simulink library "BEML_EMU_DoorsInput_Lib"  (R2019b)
settings: Solver=VariableStepAuto  StartTime=0.0  StopTime=10.0  RelTol=1e-3
undefined symbols (not defined in the file): DoorsSampleTime, DoorWinder, ElectricalSignals, EmerDoorLatched, EmerDoorOpenFault, EmergencyDoorGasSpring, EmergencyDoorHandle, EmergencyDoorMechanicalUnlocked, HasCab, InputControlStates, RampCoverLockingLever, RampHandle, RampMiddleSupport, RampWinder
libraries: simulink x128, $bdroot x8, VectorOperationsLib x1
(part 1 of 2)
settings Model: Creator=rleighton  LastModifiedBy=bnadpurohit
settings DataIOCC: ReturnWorkspaceOutputs=off
settings DebuggingCC: ArithmeticOperatorsInVariantConditions=warning
settings SFSimCC: SimUseLocalCustomCode=off  CustomCodeUndefinedFunction=UseInterfaceOnly
settings RTWCC: RTWUseLocalCustomCode=off

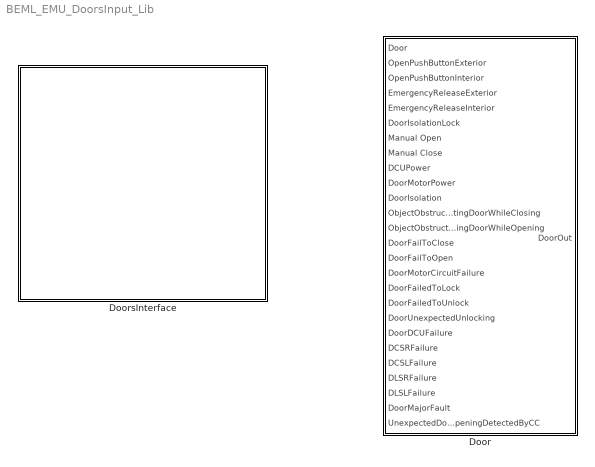
== system BEML_EMU_DoorsInput_Lib ==
  Door : Subsystem  mask{isLeft=on}
  DoorsInterface : Subsystem  SystemSampleTime=0.001

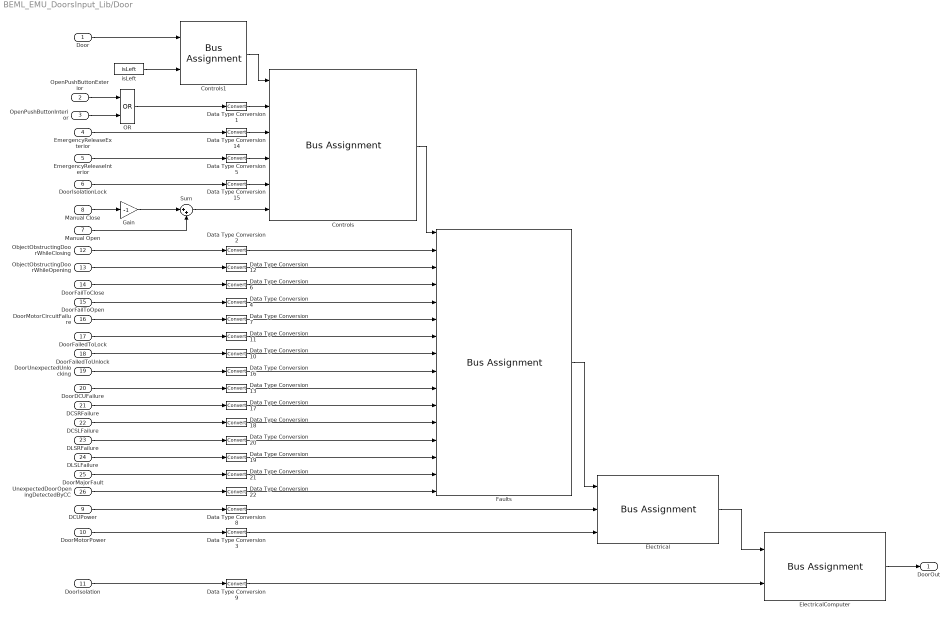
== system BEML_EMU_DoorsInput_Lib/Door ==
  Door : Inport
  OpenPushButtonExterior : Inport  Port=2
  OpenPushButtonInterior : Inport  Port=3
  EmergencyReleaseExterior : Inport  Port=4
  EmergencyReleaseInterior : Inport  Port=5
  DoorIsolationLock : Inport  Port=6
  Manual Open : Inport  Port=7
  Manual Close : Inport  Port=8
  DCUPower : Inport  Port=9
  DoorMotorPower : Inport  Port=10
  DoorIsolation : Inport  Port=11
  ObjectObstructingDoorWhileClosing : Inport  Port=12
  ObjectObstructingDoorWhileOpening : Inport  Port=13
  DoorFailToClose : Inport  Port=14
  DoorFailToOpen : Inport  Port=15
  DoorMotorCircuitFailure : Inport  Port=16
  DoorFailedToLock : Inport  Port=17
  DoorFailedToUnlock : Inport  Port=18
  DoorUnexpectedUnlocking : Inport  Port=19
  DoorDCUFailure : Inport  Port=20
  DCSRFailure : Inport  Port=21
  DCSLFailure : Inport  Port=22
  DLSRFailure : Inport  Port=23
  DLSLFailure : Inport  Port=24
  DoorMajorFault : Inport  Port=25
  UnexpectedDoorOpeningDetectedByCC : Inport  Port=26
  Controls : BusAssignment  AssignedSignals=InputControlStates.LocalDoorOpenPB,InputControlStates.EmergencyAccessDevice,InputControlStates.EmergencyEgressDevice,InputControlStates.LocalDoorIsolationLock,InputControlStates.OpenCloseWidget
  Controls1 : BusAssignment  AssignedSignals=Config.isLeft
  Data Type Conversion{1..22} (22 alike) : DataTypeConversion
  Electrical : BusAssignment  AssignedSignals=ElectricalSignals.DoorControlPower,ElectricalSignals.DoorMotorPower
  ElectricalComputer : BusAssignment  AssignedSignals=ElectricalSignals.DoorIsolation
  Faults : BusAssignment  AssignedSignals=Faults.ObjectObstructingDoorWhileClosing,Faults.ObjectObstructingDoorWhileOpening,Faults.DoorFailToClose,Faults.DoorFailToOpen,Faults.DoorMotorCircuitFailure,Faults.DoorFailedToLock,Faults.DoorFailedToUnlock,Faults.DoorUnexpectedUnlocking,Faults.DoorDCUFailure,Faults.DCSRFailure,Faults.DCSLFailure,Faults.DLSRFailure,Faults.DLSLFailure,Faults.DoorMajorFault,Faults.UnexpectedDoorOpeningDetectedByCC
  Gain : Gain  Gain=-1
  OR : Logic  Operator=OR  AllPortsSameDT=off  OutDataTypeStr=boolean
  Sum : Sum  Inputs=|++
  isLeft : Constant  Value=isLeft
  "DoorOut " : Outport  VectorParamsAs1DForOutWhenUnconnected=off
  wires:
  Data Type Conversion22/1 -> Faults/16
  UnexpectedDoorOpeningDetectedByCC/1 -> Data Type Conversion22/1
  OR/1 -> Data Type Conversion1/1
  OpenPushButtonInterior/1 -> OR/2
  DoorIsolationLock/1 -> Data Type Conversion15/1
  EmergencyReleaseExterior/1 -> Data Type Conversion14/1
  ObjectObstructingDoorWhileOpening/1 -> Data Type Conversion12/1
  Data Type Conversion12/1 -> Faults/3
  Data Type Conversion8/1 -> Electrical/2
  Data Type Conversion1/1 -> Controls/2
  OpenPushButtonExterior/1 -> OR/1
  Electrical/1 -> ElectricalComputer/1
  Sum/1 -> Controls/6
  ObjectObstructingDoorWhileClosing/1 -> Data Type Conversion2/1
  Data Type Conversion2/1 -> Faults/2
  Faults/1 -> Electrical/1
  Controls/1 -> Faults/1
  Door/1 -> Controls1/1
  Controls1/1 -> Controls/1
  isLeft/1 -> Controls1/2
  Manual Close/1 -> Gain/1
  Gain/1 -> Sum/1
  Manual Open/1 -> Sum/2
  DCUPower/1 -> Data Type Conversion8/1
  Data Type Conversion5/1 -> Controls/4
  Data Type Conversion15/1 -> Controls/5
  Data Type Conversion14/1 -> Controls/3
  DoorMotorPower/1 -> Data Type Conversion3/1
  Data Type Conversion3/1 -> Electrical/3
  Data Type Conversion6/1 -> Faults/4
  DoorFailToClose/1 -> Data Type Conversion6/1
  Data Type Conversion4/1 -> Faults/5
  DoorFailToOpen/1 -> Data Type Conversion4/1
  DoorMotorCircuitFailure/1 -> Data Type Conversion7/1
  Data Type Conversion7/1 -> Faults/6
  ElectricalComputer/1 -> "DoorOut "/1
  Data Type Conversion9/1 -> ElectricalComputer/2
  DoorIsolation/1 -> Data Type Conversion9/1
  Data Type Conversion17/1 -> Faults/11
  DCSRFailure/1 -> Data Type Conversion17/1
  DoorDCUFailure/1 -> Data Type Conversion13/1
  Data Type Conversion13/1 -> Faults/10
  DoorUnexpectedUnlocking/1 -> Data Type Conversion16/1
  Data Type Conversion16/1 -> Faults/9
  Data Type Conversion11/1 -> Faults/7
  DoorFailedToLock/1 -> Data Type Conversion11/1
  Data Type Conversion10/1 -> Faults/8
  DoorFailedToUnlock/1 -> Data Type Conversion10/1
  DCSLFailure/1 -> Data Type Conversion18/1
  Data Type Conversion18/1 -> Faults/12
  Data Type Conversion20/1 -> Faults/13
  DLSRFailure/1 -> Data Type Conversion20/1
  Data Type Conversion19/1 -> Faults/14
  DLSLFailure/1 -> Data Type Conversion19/1
  DoorMajorFault/1 -> Data Type Conversion21/1
  Data Type Conversion21/1 -> Faults/15
  EmergencyReleaseInterior/1 -> Data Type Conversion5/1

== system BEML_EMU_DoorsInput_Lib/DoorsInterface ==
  DoorsInputAdapter : Subsystem  TreatAsAtomicUnit=on  SystemSampleTime=DoorsSampleTime

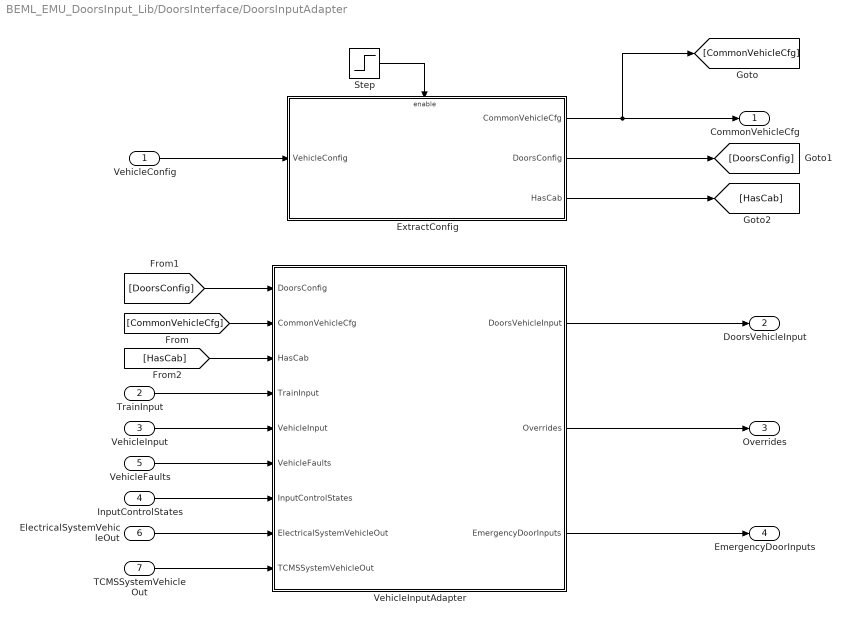
== system BEML_EMU_DoorsInput_Lib/DoorsInterface/DoorsInputAdapter ==
  VehicleConfig : Inport  SampleTime=0.05
  TrainInput : Inport  Port=2  SampleTime=0.05
  VehicleInput : Inport  Port=3  SampleTime=0.05
  InputControlStates : Inport  Port=4  SampleTime=0.05
  VehicleFaults : Inport  Port=5  SampleTime=0.05
  ElectricalSystemVehicleOut : Inport  Port=6  SampleTime=0.05
  TCMSSystemVehicleOut : Inport  Port=7  SampleTime=0.05
  ExtractConfig : Subsystem
  Step : Step  Before=1  After=0
  VehicleInputAdapter : Subsystem
  CommonVehicleCfg : Outport  VectorParamsAs1DForOutWhenUnconnected=off
  DoorsVehicleInput : Outport  Port=2  VectorParamsAs1DForOutWhenUnconnected=off
  Overrides : Outport  Port=3  VectorParamsAs1DForOutWhenUnconnected=off
  EmergencyDoorInputs : Outport  Port=4  VectorParamsAs1DForOutWhenUnconnected=off
  wires:
  [HasCab] -> VehicleInputAdapter/3(HasCab)
  ExtractConfig/3(HasCab) -> [HasCab]
  [CommonVehicleCfg] -> VehicleInputAdapter/2(CommonVehicleCfg)
  VehicleInputAdapter/3(EmergencyDoorInputs) -> EmergencyDoorInputs/1
  [DoorsConfig] -> VehicleInputAdapter/1(DoorsConfig)
  ExtractConfig/2(DoorsConfig) -> [DoorsConfig]
  InputControlStates/1 -> VehicleInputAdapter/7(InputControlStates)
  VehicleConfig/1 -> ExtractConfig/1(VehicleConfig)
  VehicleFaults/1 -> VehicleInputAdapter/6(VehicleFaults)
  TrainInput/1 -> VehicleInputAdapter/4(TrainInput)
  VehicleInput/1 -> VehicleInputAdapter/5(VehicleInput)
  ElectricalSystemVehicleOut/1 -> VehicleInputAdapter/8(ElectricalSystemVehicleOut)
  TCMSSystemVehicleOut/1 -> VehicleInputAdapter/9(TCMSSystemVehicleOut)
  ExtractConfig/1(CommonVehicleCfg) -> [CommonVehicleCfg], CommonVehicleCfg/1
  Step/1 -> ExtractConfig/Enable
  VehicleInputAdapter/1(DoorsVehicleInput) -> DoorsVehicleInput/1
  VehicleInputAdapter/2(Overrides) -> Overrides/1

== system BEML_EMU_DoorsInput_Lib/DoorsInterface/DoorsInputAdapter/ExtractConfig ==
  VehicleConfig : Inport
  Enable : EnablePort
  ExtractConfig : Subsystem
  CommonVehicleCfg : Outport  VectorParamsAs1DForOutWhenUnconnected=off
  DoorsConfig : Outport  Port=2  VectorParamsAs1DForOutWhenUnconnected=off
  HasCab : Outport  Port=3  VectorParamsAs1DForOutWhenUnconnected=off
  wires:
  ExtractConfig/3(HasCab) -> HasCab/1
  ExtractConfig/2(DoorsConfig) -> DoorsConfig/1
  ExtractConfig/1(CommonVehicleConfig) -> CommonVehicleCfg/1
  VehicleConfig/1 -> ExtractConfig/1(VehicleConfig)

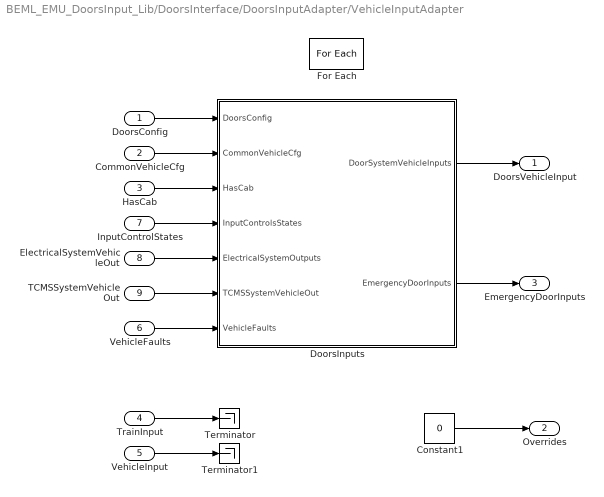
== system BEML_EMU_DoorsInput_Lib/DoorsInterface/DoorsInputAdapter/VehicleInputAdapter ==
  DoorsConfig : Inport  Partition=on  PartitionDimension=1  PartitionWidth=1  PartitionOffset=0
  CommonVehicleCfg : Inport  Port=2  Partition=on  PartitionDimension=1  PartitionWidth=1  PartitionOffset=0
  HasCab : Inport  Port=3  Partition=on  PartitionDimension=1  PartitionWidth=1  PartitionOffset=0
  TrainInput : Inport  Port=4
  VehicleInput : Inport  Port=5  Partition=on  PartitionDimension=1  PartitionWidth=1  PartitionOffset=0
  VehicleFaults : Inport  Port=6  Partition=on  PartitionDimension=1  PartitionWidth=1  PartitionOffset=0
  InputControlStates : Inport  Port=7  Partition=on  PartitionDimension=1  PartitionWidth=1  PartitionOffset=0
  ElectricalSystemVehicleOut : Inport  Port=8  Partition=on  PartitionDimension=1  PartitionWidth=1  PartitionOffset=0
  TCMSSystemVehicleOut : Inport  Port=9  Partition=on  PartitionDimension=1  PartitionWidth=1  PartitionOffset=0
  Constant1 : Constant  Value=0  OutDataTypeStr=Bus: BD_DoorSystem_In_Overrides
  DoorsInputs : Subsystem
  For Each : ForEach  DisableCoverage=on
  Terminator : Terminator
  Terminator1 : Terminator
  DoorsVehicleInput : Outport  ConcatenationDimension=1  VectorParamsAs1DForOutWhenUnconnected=off
  Overrides : Outport  Port=2  ConcatenationDimension=1  VectorParamsAs1DForOutWhenUnconnected=off
  EmergencyDoorInputs : Outport  Port=3  ConcatenationDimension=1  VectorParamsAs1DForOutWhenUnconnected=off
  wires:
  HasCab/1 -> DoorsInputs/3(HasCab)
  CommonVehicleCfg/1 -> DoorsInputs/2(CommonVehicleCfg)
  DoorsInputs/2(EmergencyDoorInputs) -> EmergencyDoorInputs/1
  DoorsConfig/1 -> DoorsInputs/1(DoorsConfig)
  InputControlStates/1 -> DoorsInputs/4(InputControlsStates)
  Constant1/1 -> Overrides/1
  DoorsInputs/1(DoorSystemVehicleInputs) -> DoorsVehicleInput/1
  TCMSSystemVehicleOut/1 -> DoorsInputs/6(TCMSSystemVehicleOut)
  ElectricalSystemVehicleOut/1 -> DoorsInputs/5(ElectricalSystemOutputs)
  VehicleFaults/1 -> DoorsInputs/7(VehicleFaults)
  VehicleInput/1 -> Terminator1/1
  TrainInput/1 -> Terminator/1

== system BEML_EMU_DoorsInput_Lib/DoorsInterface/DoorsInputAdapter/ExtractConfig/ExtractConfig ==
  VehicleConfig : Inport  Partition=on  PartitionDimension=1  PartitionWidth=1  PartitionOffset=0  BusOutputAsStruct=on
  Bus Selector : BusSelector  OutputSignals=Common,Doors,Equipment.HasCab
  For Each : ForEach  DisableCoverage=on
  CommonVehicleConfig : Outport  ConcatenationDimension=1  VectorParamsAs1DForOutWhenUnconnected=off
  DoorsConfig : Outport  Port=2  ConcatenationDimension=1  VectorParamsAs1DForOutWhenUnconnected=off
  HasCab : Outport  Port=3  ConcatenationDimension=1  VectorParamsAs1DForOutWhenUnconnected=off
  wires:
  Bus Selector/3 -> HasCab/1  "<HasCab>"
  Bus Selector/2 -> DoorsConfig/1  "<Doors>"
  VehicleConfig/1 -> Bus Selector/1
  Bus Selector/1 -> CommonVehicleConfig/1  "<Common>"

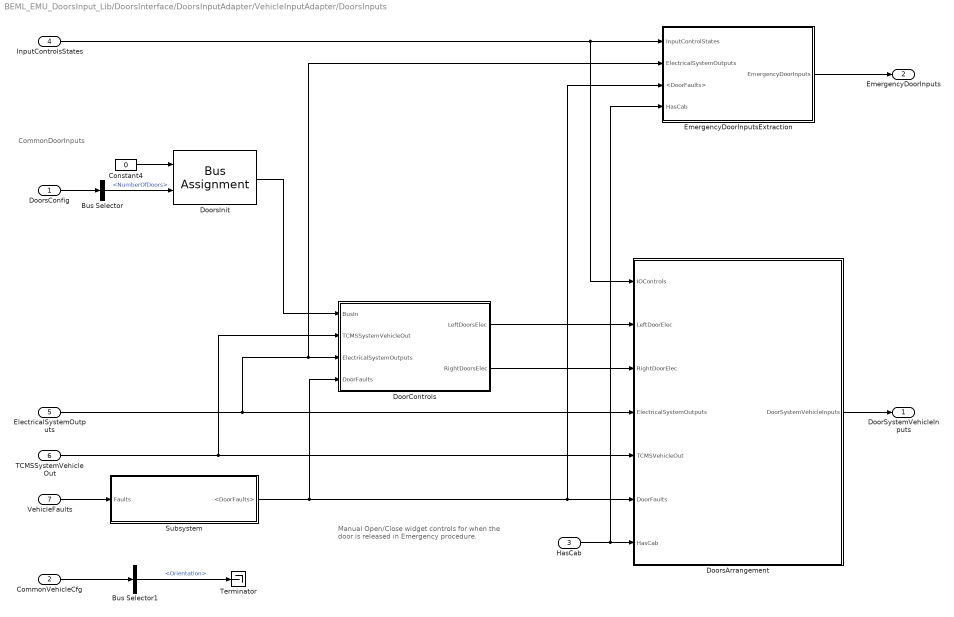
== system BEML_EMU_DoorsInput_Lib/DoorsInterface/DoorsInputAdapter/VehicleInputAdapter/DoorsInputs ==
  note: CommonDoorInputs
  note: Manual Open/Close widget controls for when the door is released in Emergency procedure.
  DoorsConfig : Inport
  CommonVehicleCfg : Inport  Port=2
  HasCab : Inport  Port=3
  InputControlsStates : Inport  Port=4
  ElectricalSystemOutputs : Inport  Port=5
  TCMSSystemVehicleOut : Inport  Port=6
  VehicleFaults : Inport  Port=7
  Bus Selector : BusSelector  OutputSignals=NumberOfDoors
  Bus Selector1 : BusSelector  OutputSignals=Orientation
  Constant4 : Constant  Value=0  OutDataTypeStr=Bus: BD_DoorSystem_In_Door  SampleTime=-1
  DoorControls : Subsystem
  DoorsArrangement : Subsystem
  DoorsInit : BusAssignment  AssignedSignals=Config.NumberOfDoors
  EmergencyDoorInputsExtraction : Subsystem
  Subsystem : Subsystem
  Terminator : Terminator
  DoorSystemVehicleInputs : Outport  VectorParamsAs1DForOutWhenUnconnected=off
  EmergencyDoorInputs : Outport  Port=2  VectorParamsAs1DForOutWhenUnconnected=off
  wires:
  HasCab/1 -> DoorsArrangement/7(HasCab), EmergencyDoorInputsExtraction/4(HasCab)
  DoorControls/2(RightDoorsElec) -> DoorsArrangement/3(RightDoorElec)
  Bus Selector1/1 -> Terminator/1  "<Orientation>"
  Subsystem/1(<DoorFaults>) -> DoorsArrangement/6(DoorFaults), EmergencyDoorInputsExtraction/3(<DoorFaults>), DoorControls/4(DoorFaults)
  VehicleFaults/1 -> Subsystem/1(Faults)
  CommonVehicleCfg/1 -> Bus Selector1/1
  EmergencyDoorInputsExtraction/1(EmergencyDoorInputs) -> EmergencyDoorInputs/1
  InputControlsStates/1 -> DoorsArrangement/1(IOControls), EmergencyDoorInputsExtraction/1(InputControlStates)
  ElectricalSystemOutputs/1 -> DoorsArrangement/4(ElectricalSystemOutputs), DoorControls/3(ElectricalSystemOutputs), EmergencyDoorInputsExtraction/2(ElectricalSystemOutputs)
  DoorsConfig/1 -> Bus Selector/1
  DoorControls/1(LeftDoorsElec) -> DoorsArrangement/2(LeftDoorElec)
  TCMSSystemVehicleOut/1 -> DoorsArrangement/5(TCMSVehicleOut), DoorControls/2(TCMSSystemVehicleOut)
  Bus Selector/1 -> DoorsInit/2  "<NumberOfDoors>"
  DoorsInit/1 -> DoorControls/1(BusIn)
  DoorsArrangement/1(DoorSystemVehicleInputs) -> DoorSystemVehicleInputs/1
  Constant4/1 -> DoorsInit/1

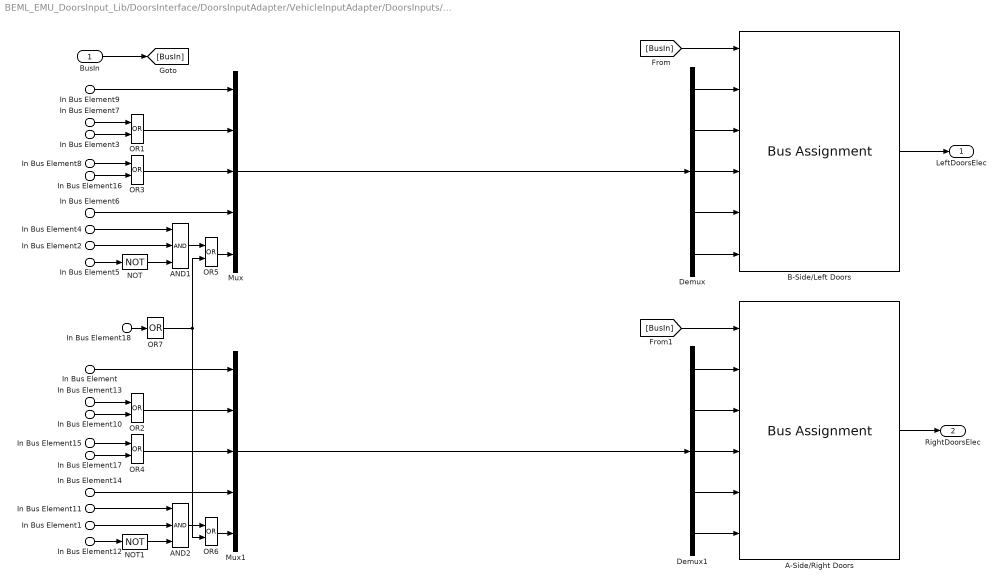
== system BEML_EMU_DoorsInput_Lib/DoorsInterface/DoorsInputAdapter/VehicleInputAdapter/DoorsInputs/DoorControls ==
  BusIn : Inport
  In Bus Element6 : Inport  Port=2  PortName=TCMSSystemVehicleOut  Element=Control.DoorSystem.LeftDoorEmergencyRelease
  In Bus Element7 : Inport  Port=2  PortName=TCMSSystemVehicleOut  Element=Control.DoorSystem.LeftSideDoorOpenRequest
  In Bus Element8 : Inport  Port=2  PortName=TCMSSystemVehicleOut  Element=Control.DoorSystem.LeftSideDoorCloseRequest
  In Bus Element9 : Inport  Port=2  PortName=TCMSSystemVehicleOut  Element=Control.DoorSystem.LeftSideDoorRelease
  In Bus Element : Inport  Port=2  PortName=TCMSSystemVehicleOut  Element=Control.DoorSystem.RightSideDoorRelease
  In Bus Element13 : Inport  Port=2  PortName=TCMSSystemVehicleOut  Element=Control.DoorSystem.RightSideDoorOpenRequest
  In Bus Element14 : Inport  Port=2  PortName=TCMSSystemVehicleOut  Element=Control.DoorSystem.RightDoorEmergencyRelease
  In Bus Element15 : Inport  Port=2  PortName=TCMSSystemVehicleOut  Element=Control.DoorSystem.RightSideDoorCloseRequest
  In Bus Element2 : Inport  Port=3  PortName=ElectricalSystemOutputs  Element=Doors.ZeroSpeed
  In Bus Element1 : Inport  Port=3  PortName=ElectricalSystemOutputs  Element=Doors.ZeroSpeed
  In Bus Element3 : Inport  Port=3  PortName=ElectricalSystemOutputs  Element=Doors.LeftDoorOpenCmdInLimpHome
  In Bus Element4 : Inport  Port=3  PortName=ElectricalSystemOutputs  Element=Doors.LeftDoorEnable
  In Bus Element5 : Inport  Port=3  PortName=ElectricalSystemOutputs  Element=Doors.LeftHoldDoorClose
  In Bus Element10 : Inport  Port=3  PortName=ElectricalSystemOutputs  Element=Doors.RightDoorOpenCmdInLimpHome
  In Bus Element11 : Inport  Port=3  PortName=ElectricalSystemOutputs  Element=Doors.RightDoorEnable
  In Bus Element12 : Inport  Port=3  PortName=ElectricalSystemOutputs  Element=Doors.RightHoldDoorClose
  In Bus Element16 : Inport  Port=3  PortName=ElectricalSystemOutputs  Element=Doors.LeftDoorClose
  In Bus Element17 : Inport  Port=3  PortName=ElectricalSystemOutputs  Element=Doors.RightDoorClose
  In Bus Element18 : Inport  Port=4  PortName=DoorFaults  Element=UnexpectedDoorOpeningDetectedByCC
  A-Side/Right Doors : BusAssignment  AssignedSignals=ElectricalSignals.DoorRelease,ElectricalSignals.DoorOpen,ElectricalSignals.DoorClose,ElectricalSignals.DoorEmergencyRelease,ElectricalSignals.DoorEnable
  AND1 : Logic  Inputs=3  AllPortsSameDT=off  OutDataTypeStr=boolean
  AND2 : Logic  Inputs=3  AllPortsSameDT=off  OutDataTypeStr=boolean
  B-Side/Left Doors : BusAssignment  AssignedSignals=ElectricalSignals.DoorRelease,ElectricalSignals.DoorOpen,ElectricalSignals.DoorClose,ElectricalSignals.DoorEmergencyRelease,ElectricalSignals.DoorEnable
  Demux : Demux  Outputs=5
  Demux1 : Demux  Outputs=5
  Mux : Mux  Inputs=5
  Mux1 : Mux  Inputs=5
  NOT : Logic  Operator=NOT  AllPortsSameDT=off  OutDataTypeStr=boolean
  NOT1 : Logic  Operator=NOT  AllPortsSameDT=off  OutDataTypeStr=boolean
  OR{1..6} (6 alike) : Logic  Operator=OR  AllPortsSameDT=off  OutDataTypeStr=boolean
  OR7 : Logic  Operator=OR  Inputs=1  AllPortsSameDT=off  OutDataTypeStr=boolean
  LeftDoorsElec : Outport
  RightDoorsElec : Outport  Port=2
  wires:
  OR7/1 -> OR5/2, OR6/2
  In Bus Element18/1 -> OR7/1
  OR5/1 -> Mux/5
  OR6/1 -> Mux1/5
  NOT1/1 -> AND2/3
  NOT/1 -> AND1/3
  In Bus Element5/1 -> NOT/1
  In Bus Element12/1 -> NOT1/1
  In Bus Element17/1 -> OR4/2
  In Bus Element15/1 -> OR4/1
  In Bus Element16/1 -> OR3/2
  In Bus Element8/1 -> OR3/1
  Demux1/5 -> A-Side/Right Doors/6
  Demux1/4 -> A-Side/Right Doors/5
  Demux1/3 -> A-Side/Right Doors/4
  Demux1/2 -> A-Side/Right Doors/3
  Demux1/1 -> A-Side/Right Doors/2
  Demux/5 -> B-Side/Left Doors/6
  Demux/4 -> B-Side/Left Doors/5
  Demux/3 -> B-Side/Left Doors/4
  Demux/2 -> B-Side/Left Doors/3
  Demux/1 -> B-Side/Left Doors/2
  Mux1/1 -> Demux1/1
  Mux/1 -> Demux/1
  [BusIn] -> B-Side/Left Doors/1
  BusIn/1 -> [BusIn]
  In Bus Element/1 -> Mux1/1
  In Bus Element11/1 -> AND2/1
  In Bus Element13/1 -> OR2/1
  In Bus Element10/1 -> OR2/2
  A-Side/Right Doors/1 -> RightDoorsElec/1
  OR4/1 -> Mux1/3
  [BusIn] -> A-Side/Right Doors/1
  In Bus Element1/1 -> AND2/2
  AND2/1 -> OR6/1
  OR2/1 -> Mux1/2
  In Bus Element14/1 -> Mux1/4
  In Bus Element2/1 -> AND1/2
  In Bus Element4/1 -> AND1/1
  AND1/1 -> OR5/1
  In Bus Element3/1 -> OR1/2
  In Bus Element7/1 -> OR1/1
  OR1/1 -> Mux/2
  OR3/1 -> Mux/3
  In Bus Element9/1 -> Mux/1
  In Bus Element6/1 -> Mux/4
  B-Side/Left Doors/1 -> LeftDoorsElec/1

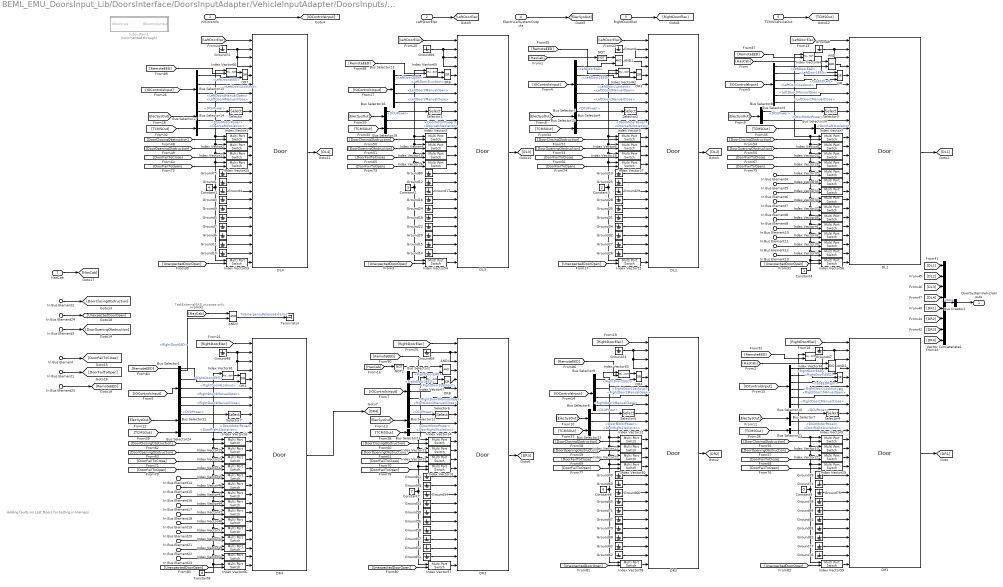
== system BEML_EMU_DoorsInput_Lib/DoorsInterface/DoorsInputAdapter/VehicleInputAdapter/DoorsInputs/DoorsArrangement ==
  note: Adding faults on Last Doors for testing in Harness
  note: TestExternalEAD purpose only
  IOControls : Inport
  LeftDoorElec : Inport  Port=2
  RightDoorElec : Inport  Port=3
  ElectricalSystemOutputs : Inport  Port=4
  TCMSVehicleOut : Inport  Port=5
  In Bus Element2 : Inport  Port=6  PortName=DoorFaults  Element=ObjectObstructingDoorWhileClosing
  In Bus Element3 : Inport  Port=6  PortName=DoorFaults  Element=ObjectObstructingDoorWhileOpening
  In Bus Element : Inport  Port=6  PortName=DoorFaults  Element=DoorFailToClose
  In Bus Element1 : Inport  Port=6  PortName=DoorFaults  Element=DoorFailToOpen
  In Bus Element4 : Inport  Port=6  PortName=DoorFaults  Element=DoorMotorCircuitFailure
  In Bus Element14 : Inport  Port=6  PortName=DoorFaults  Element=DoorMotorCircuitFailure
  In Bus Element5 : Inport  Port=6  PortName=DoorFaults  Element=DoorFailedToLock
  In Bus Element15 : Inport  Port=6  PortName=DoorFaults  Element=DoorFailedToLock
  In Bus Element6 : Inport  Port=6  PortName=DoorFaults  Element=DoorFailedToUnlock
  In Bus Element16 : Inport  Port=6  PortName=DoorFaults  Element=DoorFailedToUnlock
  In Bus Element7 : Inport  Port=6  PortName=DoorFaults  Element=DoorUnexpectedUnlocking
  In Bus Element17 : Inport  Port=6  PortName=DoorFaults  Element=DoorUnexpectedUnlocking
  In Bus Element8 : Inport  Port=6  PortName=DoorFaults  Element=DoorDCUFailure
  In Bus Element18 : Inport  Port=6  PortName=DoorFaults  Element=DoorDCUFailure
  In Bus Element9 : Inport  Port=6  PortName=DoorFaults  Element=DCSRFailure
  In Bus Element19 : Inport  Port=6  PortName=DoorFaults  Element=DCSRFailure
  In Bus Element10 : Inport  Port=6  PortName=DoorFaults  Element=DCSLFailure
  In Bus Element20 : Inport  Port=6  PortName=DoorFaults  Element=DCSLFailure
  In Bus Element11 : Inport  Port=6  PortName=DoorFaults  Element=DLSRFailure
  In Bus Element21 : Inport  Port=6  PortName=DoorFaults  Element=DLSRFailure
  In Bus Element12 : Inport  Port=6  PortName=DoorFaults  Element=DLSLFailure
  In Bus Element22 : Inport  Port=6  PortName=DoorFaults  Element=DLSLFailure
  In Bus Element13 : Inport  Port=6  PortName=DoorFaults  Element=DoorMajorFault
  In Bus Element23 : Inport  Port=6  PortName=DoorFaults  Element=DoorMajorFault
  In Bus Element24 : Inport  Port=6  PortName=DoorFaults  Element=UnexpectedDoorOpeningDetectedByCC
  In Bus Element25 : Inport  Port=6  PortName=DoorFaults  Element=RemoteEED
  HasCab : Inport  Port=7
  AND{,1..4} (5 alike) : Logic  AllPortsSameDT=off  OutDataTypeStr=boolean
  Bus Creator1 : BusCreator  Inputs='Doors'  OutDataTypeStr=Bus: BD_DoorSystem_In_Vehicle  NonVirtualBus=on
  Bus Selector1 : BusSelector  OutputSignals=RightDoorEAD,RightDoor4EED,RightDoor4Lockout,RightDoor4ManualOpen,RightDoor4ManualClose
  Bus Selector10 : BusSelector  OutputSignals=RightDoorEAD,RightDoor1EED,CabEEDRight,RightDoor1Lockout,RightDoor1ManualOpen,RightDoor1ManualClose
  Bus Selector{4,6..8,11..12,14,16} (8 alike) : BusSelector  OutputSignals=Doors.DCUPower,Doors.DoorMotorPower
  Bus Selector13 : BusSelector  OutputSignals=LeftDoor3EED,LeftDoor3Lockout,LeftDoor3ManualOpen,LeftDoor3ManualClose
  Bus Selector15 : BusSelector  OutputSignals=LeftDoor4EED,LeftDoor4Lockout,LeftDoor4ManualOpen,LeftDoor4ManualClose
  Bus Selector17 : BusSelector  OutputSignals=Control.DoorSystem.DoorLeft4Isolation
  Bus Selector18 : BusSelector  OutputSignals=Control.DoorSystem.DoorLeft3Isolation
  Bus Selector19 : BusSelector  OutputSignals=Control.DoorSystem.DoorLeft2Isolation
  Bus Selector2 : BusSelector  OutputSignals=RightDoorEAD,RightDoor3EED,RightDoor3Lockout,RightDoor3ManualOpen,RightDoor3ManualClose
  Bus Selector20 : BusSelector  OutputSignals=Control.DoorSystem.DoorLeft1Isolation
  Bus Selector21 : BusSelector  OutputSignals=Control.DoorSystem.DoorRight1Isolation
  Bus Selector22 : BusSelector  OutputSignals=Control.DoorSystem.DoorRight2Isolation
  Bus Selector23 : BusSelector  OutputSignals=Control.DoorSystem.DoorRight3Isolation
  Bus Selector24 : BusSelector  OutputSignals=Control.DoorSystem.DoorRight4Isolation
  Bus Selector3 : BusSelector  OutputSignals=LeftDoorEAD,LeftDoor1EED,CabEEDLeft,LeftDoor1Lockout,LeftDoor1ManualOpen,LeftDoor1ManualClose
  Bus Selector5 : BusSelector  OutputSignals=LeftDoorEAD,LeftDoor2EED,LeftDoor2Lockout,LeftDoor2ManualOpen,LeftDoor2ManualClose
  Bus Selector9 : BusSelector  OutputSignals=RightDoor2EED,RightDoor2Lockout,RightDoor2ManualOpen,RightDoor2ManualClose
  Constant1 : Constant  Value=4
  Constant2 : Constant  Value=3
  Constant3 : Constant  Value=2
  Constant4 : Constant
  Constant5 : Constant  Value=5
  Constant6 : Constant  Value=6
  Constant7 : Constant  Value=7
  Constant8 : Constant  Value=8
  DL{1..4} (4 alike) : $bdroot/Door  isLeft=on
  DR{1..4} (4 alike) : $bdroot/Door  isLeft=off
  Ground{,1,3..17,19..20,22..32,34..35,39,47..49,51..54,56..63,65..72,74..84,94} (68 alike) : Ground
  Index Vector{1..68} (68 alike) : MultiPortSwitch  Inputs=1
  NOT : Logic  Operator=NOT  AllPortsSameDT=off  OutDataTypeStr=boolean
  NOT2 : Logic  Operator=NOT  AllPortsSameDT=off  OutDataTypeStr=boolean
  OR : Logic  Operator=OR  Inputs=3  AllPortsSameDT=off  OutDataTypeStr=boolean
  OR1 : Logic  Operator=OR  Inputs=3  AllPortsSameDT=off  OutDataTypeStr=boolean
  OR{2..4,6..8} (6 alike) : Logic  Operator=OR  AllPortsSameDT=off  OutDataTypeStr=boolean
  Selector : Selector  InputPortWidth=MaxDoors  IndexOptions=Index vector (dialog)  Indices=4  OutputSizes=1
  Selector1 : Selector  InputPortWidth=MaxDoors  IndexOptions=Index vector (dialog)  Indices=3  OutputSizes=1
  Selector2 : Selector  InputPortWidth=MaxDoors  IndexOptions=Index vector (dialog)  Indices=2  OutputSizes=1
  Selector3 : Selector  InputPortWidth=MaxDoors  IndexOptions=Index vector (dialog)  Indices=1  OutputSizes=1
  Selector4 : Selector  InputPortWidth=MaxDoors  IndexOptions=Index vector (dialog)  Indices=5  OutputSizes=1
  Selector5 : Selector  InputPortWidth=MaxDoors  IndexOptions=Index vector (dialog)  Indices=6  OutputSizes=1
  Selector6 : Selector  InputPortWidth=MaxDoors  IndexOptions=Index vector (dialog)  Indices=7  OutputSizes=1
  Selector7 : Selector  InputPortWidth=MaxDoors  IndexOptions=Index vector (dialog)  Indices=8  OutputSizes=1
  Subsystem1 : Subsystem  Commented=through
  Terminator : Terminator
  Vector Concatenate1 : Concatenate  NumInputs=8
  DoorSystemVehicleInputs : Outport
  wires:
  AND3/1 -> Terminator/1  "ToEmergencyReleaseExterior"
  Bus Selector1/1 -> AND3/2  "<RightDoorEAD>"
  [HasCab] -> AND3/1
  OR7/1 -> DL4/5
  OR6/1 -> DL3/5
  [RemoteEED] -> Index Vector65/2
  Index Vector65/1 -> OR6/1
  Index Vector66/1 -> OR7/1
  [RemoteEED] -> Index Vector66/2
  OR3/1 -> DL2/5
  Index Vector68/1 -> OR1/1
  [RemoteEED] -> Index Vector68/2
  OR4/1 -> DR2/5
  OR8/1 -> DR3/5
  Index Vector67/1 -> OR8/1
  [RemoteEED] -> Index Vector67/2
  [RemoteEED] -> Index Vector64/2
  Index Vector64/1 -> OR/1
  Index Vector63/1 -> OR4/1
  [RemoteEED] -> Index Vector63/2
  [RemoteEED] -> Index Vector62/2
  Index Vector62/1 -> OR3/1
  OR2/1 -> DR4/5
  Index Vector61/1 -> OR2/1
  [RemoteEED] -> Index Vector61/2
  In Bus Element25/1 -> [RemoteEED]
  Selector7/1 -> DR4/9
  Selector6/1 -> DR3/9
  Selector5/1 -> DR2/9
  Selector4/1 -> DR1/9
  Selector3/1 -> DL1/9
  Selector2/1 -> DL2/9
  Selector1/1 -> DL3/9
  Selector/1 -> DL4/9
  Index Vector60/1 -> DR4/26
  [UnexpectedDoorOpen] -> Index Vector60/2
  Index Vector59/1 -> DR1/26
  [UnexpectedDoorOpen] -> Index Vector59/2
  Constant5/1 -> Index Vector59/1, Index Vector29/1, Index Vector21/1, Index Vector10/1, Index Vector68/1, Index Vector9/1
  Constant6/1 -> Index Vector58/1, Index Vector30/1, Index Vector22/1, Index Vector11/1, Index Vector63/1, Index Vector12/1
  [UnexpectedDoorOpen] -> Index Vector58/2
  Index Vector58/1 -> DR2/26
  Index Vector57/1 -> DR3/26
  [UnexpectedDoorOpen] -> Index Vector57/2
  Constant7/1 -> Index Vector57/1, Index Vector31/1, Index Vector23/1, Index Vector13/1, Index Vector14/1, Index Vector67/1
  Index Vector56/1 -> DL1/26
  [UnexpectedDoorOpen] -> Index Vector56/2
  [UnexpectedDoorOpen] -> Index Vector55/2
  Constant3/1 -> Index Vector55/1, Index Vector27/1, Index Vector19/1, Index Vector6/1, Index Vector62/1, Index Vector5/1
  Index Vector55/1 -> DL2/26
  In Bus Element24/1 -> [UnexpectedDoorOpen]
  Index Vector54/1 -> DL3/26
  Constant2/1 -> Index Vector54/1, Index Vector26/1, Index Vector18/1, Index Vector4/1, Index Vector3/1, Index Vector65/1
  [UnexpectedDoorOpen] -> Index Vector54/2
  Index Vector53/1 -> DL4/26
  [UnexpectedDoorOpen] -> Index Vector53/2
  AND4/1 -> DR3/4
  [HasCab] -> NOT2/1
  NOT2/1 -> AND4/1
  Bus Selector2/1 -> AND4/2  "<RightDoorEAD>"
  AND2/1 -> DR1/4
  [HasCab] -> AND2/1
  NOT/1 -> AND1/1
  AND1/1 -> DL2/4
  [HasCab] -> NOT/1
  [HasCab] -> AND/1
  AND/1 -> DL1/4
  HasCab/1 -> [HasCab]
  Bus Selector10/3 -> OR1/3  "<CabEEDRight>"
  OR1/1 -> DR1/5
  Bus Selector3/3 -> OR/3  "<CabEEDLeft>"
  OR/1 -> DL1/5
  Index Vector50/1 -> DR4/25
  Index Vector49/1 -> DR4/24
  Index Vector52/1 -> DR4/23
  Index Vector51/1 -> DR4/22
  Index Vector48/1 -> DR4/21
  Index Vector47/1 -> DR4/20
  Index Vector44/1 -> DR4/19
  Index Vector43/1 -> DR4/18
  Index Vector46/1 -> DR4/17
  Index Vector45/1 -> DR4/16
  In Bus Element19/1 -> Index Vector48/2
  In Bus Element16/1 -> Index Vector43/2
  In Bus Element20/1 -> Index Vector51/2
  Constant8/1 -> Index Vector50/1, Index Vector49/1, Index Vector52/1, Index Vector51/1, Index Vector48/1, Index Vector47/1, Index Vector44/1, Index Vector43/1, Index Vector46/1, Index Vector45/1, Index Vector16/1, Index Vector61/1, Index Vector15/1, Index Vector24/1, Index Vector32/1, Index Vector60/1
  In Bus Element15/1 -> Index Vector46/2
  In Bus Element21/1 -> Index Vector52/2
  In Bus Element18/1 -> Index Vector47/2
  In Bus Element17/1 -> Index Vector44/2
  In Bus Element14/1 -> Index Vector45/2
  In Bus Element22/1 -> Index Vector49/2
  In Bus Element23/1 -> Index Vector50/2
  In Bus Element13/1 -> Index Vector40/2
  In Bus Element12/1 -> Index Vector39/2
  In Bus Element11/1 -> Index Vector42/2
  In Bus Element10/1 -> Index Vector41/2
  In Bus Element9/1 -> Index Vector38/2
  In Bus Element8/1 -> Index Vector37/2
  In Bus Element7/1 -> Index Vector34/2
  In Bus Element6/1 -> Index Vector33/2
  In Bus Element5/1 -> Index Vector36/2
  In Bus Element4/1 -> Index Vector35/2
  Index Vector37/1 -> DL1/20
  Index Vector38/1 -> DL1/21
  Index Vector40/1 -> DL1/25
  Index Vector39/1 -> DL1/24
  Index Vector42/1 -> DL1/23
  Index Vector41/1 -> DL1/22
  Index Vector35/1 -> DL1/16
  Index Vector36/1 -> DL1/17
  Index Vector33/1 -> DL1/18
  Index Vector34/1 -> DL1/19
  Ground77/1 -> DR1/24
  Ground76/1 -> DR1/25
  Ground84/1 -> DR1/20
  Ground81/1 -> DR1/21
  Ground82/1 -> DR1/23
  Ground83/1 -> DR1/22
  Ground79/1 -> DR1/18
  Ground78/1 -> DR1/19
  Ground74/1 -> DR1/17
  Ground60/1 -> DR2/17
  Ground65/1 -> DR2/19
  Ground66/1 -> DR2/18
  Ground70/1 -> DR2/22
  Ground68/1 -> DR2/23
  Ground67/1 -> DR2/21
  Ground71/1 -> DR2/20
  Ground62/1 -> DR2/25
  Ground63/1 -> DR2/24
  Ground52/1 -> DR3/24
  Ground51/1 -> DR3/25
  Ground59/1 -> DR3/20
  Ground56/1 -> DR3/21
  Ground57/1 -> DR3/23
  Ground58/1 -> DR3/22
  Ground54/1 -> DR3/18
  Ground53/1 -> DR3/19
  Ground49/1 -> DR3/17
  Ground27/1 -> DL2/24
  Ground26/1 -> DL2/25
  Ground35/1 -> DL2/20
  Ground31/1 -> DL2/21
  Ground32/1 -> DL2/23
  Ground34/1 -> DL2/22
  Ground29/1 -> DL2/18
  Ground28/1 -> DL2/19
  Ground25/1 -> DL2/17
  Ground12/1 -> DL3/17
  Ground16/1 -> DL3/19
  Ground17/1 -> DL3/18
  Ground22/1 -> DL3/22
  Ground20/1 -> DL3/23
  Ground19/1 -> DL3/21
  Ground24/1 -> DL3/20
  Ground14/1 -> DL3/25
  Ground15/1 -> DL3/24
  Ground11/1 -> DL4/24
  Ground10/1 -> DL4/25
  Ground9/1 -> DL4/20
  Ground5/1 -> DL4/21
  Ground6/1 -> DL4/23
  Ground7/1 -> DL4/22
  Ground4/1 -> DL4/18
  Ground3/1 -> DL4/19
  Ground1/1 -> DL4/17
  IOControls/1 -> [IOControlsInput]
  [DoorFailToOpen] -> Index Vector32/2
  Index Vector32/1 -> DR4/15
  [DoorFailToOpen] -> Index Vector31/2
  Index Vector31/1 -> DR3/15
  [DoorFailToOpen] -> Index Vector30/2
  Index Vector30/1 -> DR2/15
  [DoorFailToOpen] -> Index Vector29/2
  Index Vector29/1 -> DR1/15
  [DoorFailToOpen] -> Index Vector28/2
  Index Vector28/1 -> DL1/15
  [DoorFailToOpen] -> Index Vector27/2
  Index Vector27/1 -> DL2/15
  [DoorFailToOpen] -> Index Vector26/2
  Index Vector26/1 -> DL3/15
  [DoorFailToOpen] -> Index Vector25/2
  Index Vector25/1 -> DL4/15
  In Bus Element1/1 -> [DoorFailToOpen]
  [DoorFailToClose] -> Index Vector24/2
  Index Vector24/1 -> DR4/14
  [DoorFailToClose] -> Index Vector23/2
  Index Vector23/1 -> DR3/14
  [DoorFailToClose] -> Index Vector22/2
  Index Vector22/1 -> DR2/14
  Index Vector21/1 -> DR1/14
  [DoorFailToClose] -> Index Vector21/2
  [DoorFailToClose] -> Index Vector20/2
  [DoorFailToClose] -> Index Vector19/2
  [DoorFailToClose] -> Index Vector18/2
  [DoorFailToClose] -> Index Vector17/2
  In Bus Element/1 -> [DoorFailToClose]
  Index Vector20/1 -> DL1/14
  Index Vector19/1 -> DL2/14
  Index Vector18/1 -> DL3/14
  Index Vector17/1 -> DL4/14
  Index Vector10/1 -> DR1/13
  Index Vector9/1 -> DR1/12
  Index Vector11/1 -> DR2/13
  Index Vector12/1 -> DR2/12
  Index Vector8/1 -> DL1/13
  Index Vector7/1 -> DL1/12
  Index Vector6/1 -> DL2/13
  Index Vector5/1 -> DL2/12
  Index Vector15/1 -> DR4/13
  Index Vector16/1 -> DR4/12
  Ground80/1 -> DL3/16
  Index Vector4/1 -> DL3/13
  Index Vector3/1 -> DL3/12
  [DoorClosingObstruction] -> Index Vector16/2
  [DoorOpeningObstruction] -> Index Vector15/2
  Index Vector14/1 -> DR3/12
  Index Vector13/1 -> DR3/13
  [DoorClosingObstruction] -> Index Vector14/2
  [DoorOpeningObstruction] -> Index Vector13/2
  [DoorClosingObstruction] -> Index Vector12/2
  [DoorOpeningObstruction] -> Index Vector11/2
  [DoorOpeningObstruction] -> Index Vector10/2
  [DoorClosingObstruction] -> Index Vector9/2
  [DoorOpeningObstruction] -> Index Vector8/2
  [DoorClosingObstruction] -> Index Vector7/2
  Constant4/1 -> Index Vector7/1, Index Vector64/1, Index Vector8/1, Index Vector20/1, Index Vector28/1, Index Vector35/1, Index Vector36/1, Index Vector33/1, Index Vector34/1, Index Vector37/1, Index Vector38/1, Index Vector41/1, Index Vector42/1, Index Vector39/1, Index Vector40/1, Index Vector56/1
  [DoorClosingObstruction] -> Index Vector5/2
  [DoorOpeningObstruction] -> Index Vector6/2
  [DoorOpeningObstruction] -> Index Vector4/2
  [DoorClosingObstruction] -> Index Vector3/2
  [DoorOpeningObstruction] -> Index Vector2/2
  Index Vector2/1 -> DL4/13
  Index Vector1/1 -> DL4/12
  [DoorClosingObstruction] -> Index Vector1/2
  Constant1/1 -> Index Vector1/1, Index Vector66/1, Index Vector2/1, Index Vector17/1, Index Vector25/1, Index Vector53/1
  In Bus Element3/1 -> [DoorOpeningObstruction]
  In Bus Element2/1 -> [DoorClosingObstruction]
  [DR2] -> Vector Concatenate1/6
  [DR1] -> Vector Concatenate1/5
  [DR3] -> Vector Concatenate1/7
  [DR4] -> Vector Concatenate1/8
  [DL4] -> Vector Concatenate1/4
  [DL3] -> Vector Concatenate1/3
  [DL2] -> Vector Concatenate1/2
  [DL1] -> Vector Concatenate1/1
  Vector Concatenate1/1 -> Bus Creator1/1  "Doors"
  Bus Selector24/1 -> DR4/11  "<DoorRight4Isolation>"
  [TCMSOut] -> Bus Selector24/1
  [TCMSOut] -> Bus Selector23/1
  Bus Selector23/1 -> DR3/11  "<DoorRight3Isolation>"
  Bus Selector22/1 -> DR2/11  "<DoorRight2Isolation>"
  [TCMSOut] -> Bus Selector22/1
  [TCMSOut] -> Bus Selector21/1
  Bus Selector21/1 -> DR1/11  "<DoorRight1Isolation>"
  [TCMSOut] -> Bus Selector20/1
  Bus Selector20/1 -> DL1/11  "<DoorLeft1Isolation>"
  Bus Selector19/1 -> DL2/11  "<DoorLeft2Isolation>"
  [TCMSOut] -> Bus Selector19/1
  [TCMSOut] -> Bus Selector18/1
  Bus Selector18/1 -> DL3/11  "<DoorLeft3Isolation>"
  Bus Selector17/1 -> DL4/11  "<DoorLeft4Isolation>"
  [TCMSOut] -> Bus Selector17/1
  TCMSVehicleOut/1 -> [TCMSOut]
  Ground75/1 -> DL4/16
  Bus Selector6/1 -> Selector5/1  "<DCUPower>"
  Bus Selector8/2 -> DL1/10  "<DoorMotorPower>"
  DR2/1 -> [DR2]
  Bus Selector8/1 -> Selector3/1  "<DCUPower>"
  Bus Selector7/1 -> Selector4/1  "<DCUPower>"
  Ground8/1 -> DL1/2, DL1/3
  Bus Selector7/2 -> DR1/10  "<DoorMotorPower>"
  Ground39/1 -> DR1/16
  DR1/1 -> [DR1]
  DL2/1 -> [DL2]
  Ground23/1 -> DR2/2, DR2/3, DR2/4
  Ground/1 -> DL2/2, DL2/3
  Ground47/1 -> DR1/2, DR1/3
  Ground13/1 -> DL2/16
  DL1/1 -> [DL1]
  Ground30/1 -> DR2/16
  Bus Selector4/1 -> Selector2/1  "<DCUPower>"
  Bus Selector4/2 -> DL2/10  "<DoorMotorPower>"
  Bus Selector6/2 -> DR2/10  "<DoorMotorPower>"
  ElectricalSystemOutputs/1 -> [ElecSysOut]
  [ElecSysOut] -> Bus Selector4/1
  [ElecSysOut] -> Bus Selector8/1
  [ElecSysOut] -> Bus Selector6/1
  [ElecSysOut] -> Bus Selector7/1
  [ElecSysOut] -> Bus Selector12/1
  [ElecSysOut] -> Bus Selector11/1
  Bus Selector11/2 -> DR4/10  "<DoorMotorPower>"
  Ground69/1 -> DR3/2, DR3/3
  Ground48/1 -> DR4/2, DR4/3, DR4/4
  DR3/1 -> [DR3]
  Ground61/1 -> DR3/16
  Bus Selector12/2 -> DR3/10  "<DoorMotorPower>"
  Bus Selector12/1 -> Selector6/1  "<DCUPower>"
  DR4/1 -> [DR4]
  Bus Selector11/1 -> Selector7/1  "<DCUPower>"
  RightDoorElec/1 -> [RightDoorElec]
  [RightDoorElec] -> DR1/1
  [RightDoorElec] -> DR2/1
  [RightDoorElec] -> DR3/1
  [RightDoorElec] -> DR4/1
  LeftDoorElec/1 -> [LeftDoorElec]
  [LeftDoorElec] -> DL2/1
  [LeftDoorElec] -> DL1/1
  [LeftDoorElec] -> DL3/1
  [LeftDoorElec] -> DL4/1
  [ElecSysOut] -> Bus Selector16/1
  [ElecSysOut] -> Bus Selector14/1
  [IOControlsInput] -> Bus Selector15/1
  Bus Selector14/2 -> DL4/10  "<DoorMotorPower>"
  Bus Selector14/1 -> Selector/1  "<DCUPower>"
  DL3/1 -> [DL3]
  Ground72/1 -> DL4/2, DL4/4, DL4/3
  Bus Selector15/1 -> OR7/2  "<LeftDoor4EED>"
  DL4/1 -> [DL4]
  Bus Selector15/3 -> DL4/7  "<LeftDoor4ManualOpen>"
  Ground94/1 -> DL3/2, DL3/4, DL3/3
  Bus Selector16/1 -> Selector1/1  "<DCUPower>"
  Bus Selector16/2 -> DL3/10  "<DoorMotorPower>"
  Bus Selector15/2 -> DL4/6  "<LeftDoor4Lockout>"
  Bus Selector15/4 -> DL4/8  "<LeftDoor4ManualClose>"
  Bus Selector13/2 -> DL3/6  "<LeftDoor3Lockout>"
  Bus Selector13/1 -> OR6/2  "<LeftDoor3EED>"
  Bus Selector13/4 -> DL3/8  "<LeftDoor3ManualClose>"
  Bus Selector13/3 -> DL3/7  "<LeftDoor3ManualOpen>"
  [IOControlsInput] -> Bus Selector13/1
  Bus Selector5/2 -> OR3/2  "<LeftDoor2EED>"
  Bus Selector5/3 -> DL2/6  "<LeftDoor2Lockout>"
  Bus Selector5/5 -> DL2/8  "<LeftDoor2ManualClose>"
  Bus Selector5/4 -> DL2/7  "<LeftDoor2ManualOpen>"
  Bus Selector5/1 -> AND1/2  "<LeftDoorEAD>"
  [IOControlsInput] -> Bus Selector5/1
  Bus Selector3/2 -> OR/2  "<LeftDoor1EED>"
  Bus Selector3/6 -> DL1/8  "<LeftDoor1ManualClose>"
  Bus Selector3/4 -> DL1/6  "<LeftDoor1Lockout>"
  [IOControlsInput] -> Bus Selector3/1
  Bus Selector3/1 -> AND/2  "<LeftDoorEAD>"
  Bus Selector3/5 -> DL1/7  "<LeftDoor1ManualOpen>"
  Bus Selector1/3 -> DR4/6  "<RightDoor4Lockout>"
  Bus Selector1/2 -> OR2/2  "<RightDoor4EED>"
  Bus Selector1/5 -> DR4/8  "<RightDoor4ManualClose>"
  Bus Selector1/4 -> DR4/7  "<RightDoor4ManualOpen>"
  [IOControlsInput] -> Bus Selector1/1
  Bus Selector2/3 -> DR3/6  "<RightDoor3Lockout>"
  Bus Selector2/2 -> OR8/2  "<RightDoor3EED>"
  Bus Selector2/5 -> DR3/8  "<RightDoor3ManualClose>"
  Bus Selector2/4 -> DR3/7  "<RightDoor3ManualOpen>"
  [IOControlsInput] -> Bus Selector2/1
  Bus Selector9/2 -> DR2/6  "<RightDoor2Lockout>"
  Bus Selector9/1 -> OR4/2  "<RightDoor2EED>"
  Bus Selector9/4 -> DR2/8  "<RightDoor2ManualClose>"
  Bus Selector9/3 -> DR2/7  "<RightDoor2ManualOpen>"
  [IOControlsInput] -> Bus Selector9/1
  Bus Selector10/1 -> AND2/2  "<RightDoorEAD>"
  Bus Selector10/4 -> DR1/6  "<RightDoor1Lockout>"
  Bus Selector10/2 -> OR1/2  "<RightDoor1EED>"
  Bus Selector10/6 -> DR1/8  "<RightDoor1ManualClose>"
  Bus Selector10/5 -> DR1/7  "<RightDoor1ManualOpen>"
  [IOControlsInput] -> Bus Selector10/1
  Bus Creator1/1 -> DoorSystemVehicleInputs/1

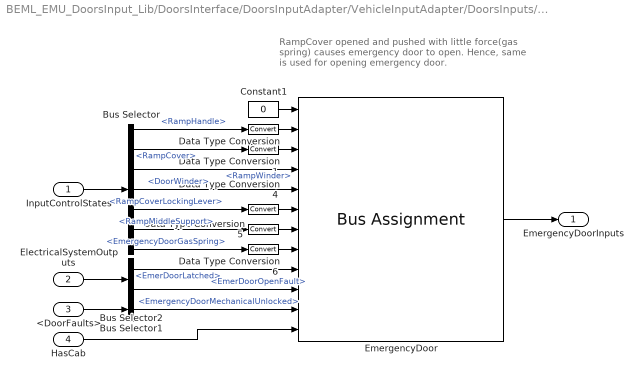
== system BEML_EMU_DoorsInput_Lib/DoorsInterface/DoorsInputAdapter/VehicleInputAdapter/DoorsInputs/EmergencyDoorInputsExtraction ==
  note: RampCover opened and pushed with little force(gas spring)
      | causes emergency door to open. Hence, same is used for opening emergency door.
  InputControlStates : Inport
  ElectricalSystemOutputs : Inport  Port=2
  <DoorFaults> : Inport  Port=3
  HasCab : Inport  Port=4
  Bus Selector : BusSelector  OutputSignals=RampHandle,RampCover,RampWinder,DoorWinder,RampCoverLockingLever,RampMiddleSupport,EmergencyDoorGasSpring
  Bus Selector1 : BusSelector  OutputSignals=EmergencyDoorMechanicalUnlocked
  Bus Selector2 : BusSelector  OutputSignals=Doors.EmerDoorLatched,Doors.EmerDoorOpenFault
  Constant1 : Constant  Value=0  OutDataTypeStr=Bus: BD_DoorSystem_In_Emergency_Door  SampleTime=-1
  Data Type Conversion{,1,4..6} (5 alike) : DataTypeConversion
  EmergencyDoor : BusAssignment  AssignedSignals=RampHandle,EmergencyDoorHandle,RampWinder,DoorWinder,RampCoverLockingLever,RampMiddleSupport,EmergencyDoorGasSpring,EmerDoorLatched,EmerDoorOpenFault,EmergencyDoorMechanicalUnlocked,HasCab
  EmergencyDoorInputs : Outport
  wires:
  HasCab/1 -> EmergencyDoor/12
  Data Type Conversion1/1 -> EmergencyDoor/3
  Data Type Conversion6/1 -> EmergencyDoor/8
  Data Type Conversion5/1 -> EmergencyDoor/7
  Bus Selector1/1 -> EmergencyDoor/11  "<EmergencyDoorMechanicalUnlocked>"
  Bus Selector2/1 -> EmergencyDoor/9  "<EmerDoorLatched>"
  Bus Selector2/2 -> EmergencyDoor/10  "<EmerDoorOpenFault>"
  Bus Selector/7 -> Data Type Conversion6/1  "<EmergencyDoorGasSpring>"
  Bus Selector/6 -> Data Type Conversion5/1  "<RampMiddleSupport>"
  Data Type Conversion4/1 -> EmergencyDoor/6
  Bus Selector/5 -> Data Type Conversion4/1  "<RampCoverLockingLever>"
  <DoorFaults>/1 -> Bus Selector1/1
  ElectricalSystemOutputs/1 -> Bus Selector2/1
  Bus Selector/4 -> EmergencyDoor/5  "<DoorWinder>"
  Bus Selector/3 -> EmergencyDoor/4  "<RampWinder>"
  Data Type Conversion/1 -> EmergencyDoor/2
  EmergencyDoor/1 -> EmergencyDoorInputs/1
  Constant1/1 -> EmergencyDoor/1
  Bus Selector/2 -> Data Type Conversion1/1  "<RampCover>"
  Bus Selector/1 -> Data Type Conversion/1  "<RampHandle>"
  InputControlStates/1 -> Bus Selector/1

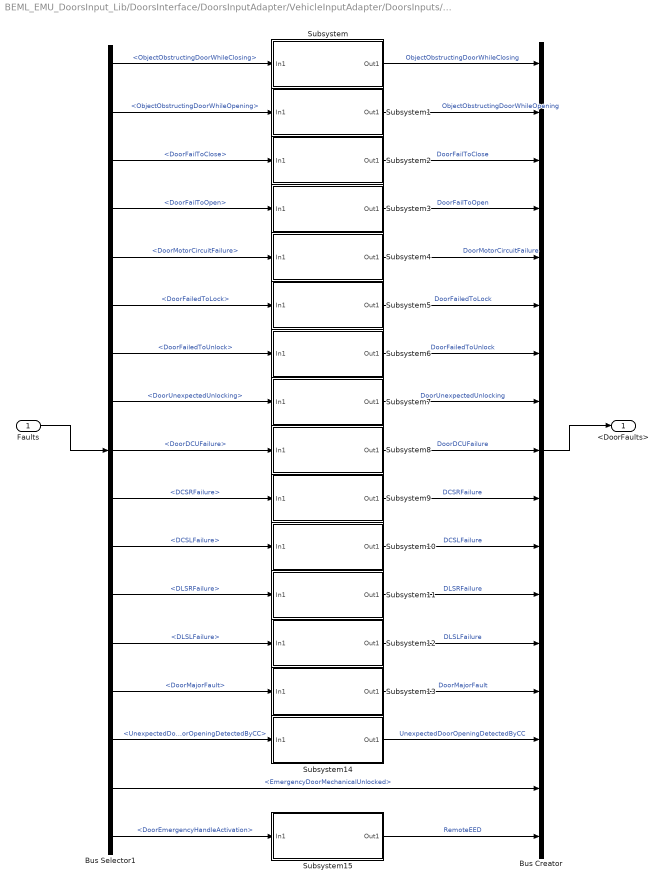
== system BEML_EMU_DoorsInput_Lib/DoorsInterface/DoorsInputAdapter/VehicleInputAdapter/DoorsInputs/Subsystem ==
  Faults : Inport
  Bus Creator : BusCreator  Inputs=17
  Bus Selector1 : BusSelector  OutputSignals=DoorFaults.ObjectObstructingDoorWhileClosing,DoorFaults.ObjectObstructingDoorWhileOpening,DoorFaults.DoorFailToClose,DoorFaults.DoorFailToOpen,DoorFaults.DoorMotorCircuitFailure,DoorFaults.DoorFailedToLock,DoorFaults.DoorFailedToUnlock,DoorFaults.DoorUnexpectedUnlocking,DoorFaults.DoorDCUFailure,DoorFaults.DCSRFailure,DoorFaults.DCSLFailure,DoorFaults.DLSRFailure,DoorFaults.DLSLFailure,DoorFaults.DoorMajorFault,DoorFaults.UnexpectedDoorOpeningDetectedByCC,DoorFaults.EmergencyDoorMechanicalUnlocked,DoorFaults.DoorEmergencyHandleActivation
  Subsystem : Subsystem
  Subsystem1 : Subsystem
  Subsystem10 : Subsystem
  Subsystem11 : Subsystem
  Subsystem12 : Subsystem
  Subsystem13 : Subsystem
  Subsystem14 : Subsystem
  Subsystem15 : Subsystem
  Subsystem2 : Subsystem
  Subsystem3 : Subsystem
  Subsystem4 : Subsystem
  Subsystem5 : Subsystem
  Subsystem6 : Subsystem
  Subsystem7 : Subsystem
  Subsystem8 : Subsystem
  Subsystem9 : Subsystem
  <DoorFaults> : Outport
  wires:
  Subsystem15/1(Out1) -> Bus Creator/17  "RemoteEED"
  Bus Selector1/17 -> Subsystem15/1(In1)  "<DoorEmergencyHandleActivation>"
  Bus Selector1/16 -> Bus Creator/16  "<EmergencyDoorMechanicalUnlocked>"
  Subsystem14/1(Out1) -> Bus Creator/15  "UnexpectedDoorOpeningDetectedByCC"
  Bus Selector1/15 -> Subsystem14/1(In1)  "<UnexpectedDoorOpeningDetectedByCC>"
  Subsystem13/1(Out1) -> Bus Creator/14  "DoorMajorFault"
  Subsystem12/1(Out1) -> Bus Creator/13  "DLSLFailure"
  Subsystem11/1(Out1) -> Bus Creator/12  "DLSRFailure"
  Subsystem10/1(Out1) -> Bus Creator/11  "DCSLFailure"
  Subsystem9/1(Out1) -> Bus Creator/10  "DCSRFailure"
  Subsystem8/1(Out1) -> Bus Creator/9  "DoorDCUFailure"
  Subsystem7/1(Out1) -> Bus Creator/8  "DoorUnexpectedUnlocking"
  Subsystem6/1(Out1) -> Bus Creator/7  "DoorFailedToUnlock"
  Subsystem5/1(Out1) -> Bus Creator/6  "DoorFailedToLock"
  Subsystem4/1(Out1) -> Bus Creator/5  "DoorMotorCircuitFailure"
  Bus Selector1/14 -> Subsystem13/1(In1)  "<DoorMajorFault>"
  Bus Selector1/13 -> Subsystem12/1(In1)  "<DLSLFailure>"
  Bus Selector1/12 -> Subsystem11/1(In1)  "<DLSRFailure>"
  Bus Selector1/11 -> Subsystem10/1(In1)  "<DCSLFailure>"
  Bus Selector1/10 -> Subsystem9/1(In1)  "<DCSRFailure>"
  Bus Selector1/9 -> Subsystem8/1(In1)  "<DoorDCUFailure>"
  Bus Selector1/8 -> Subsystem7/1(In1)  "<DoorUnexpectedUnlocking>"
  Bus Selector1/7 -> Subsystem6/1(In1)  "<DoorFailedToUnlock>"
  Bus Selector1/6 -> Subsystem5/1(In1)  "<DoorFailedToLock>"
  Bus Selector1/5 -> Subsystem4/1(In1)  "<DoorMotorCircuitFailure>"
  Subsystem3/1(Out1) -> Bus Creator/4  "DoorFailToOpen"
  Subsystem2/1(Out1) -> Bus Creator/3  "DoorFailToClose"
  Bus Creator/1 -> <DoorFaults>/1
  Bus Selector1/4 -> Subsystem3/1(In1)  "<DoorFailToOpen>"
  Bus Selector1/3 -> Subsystem2/1(In1)  "<DoorFailToClose>"
  Subsystem1/1(Out1) -> Bus Creator/2  "ObjectObstructingDoorWhileOpening"
  Subsystem/1(Out1) -> Bus Creator/1  "ObjectObstructingDoorWhileClosing"
  Bus Selector1/2 -> Subsystem1/1(In1)  "<ObjectObstructingDoorWhileOpening>"
  Bus Selector1/1 -> Subsystem/1(In1)  "<ObjectObstructingDoorWhileClosing>"
  Faults/1 -> Bus Selector1/1
